simulink model "fig2"  (R2016b)
settings: Solver=VariableStepAuto  StartTime=0.0  StopTime=70  RelTol=1e-3
values from neighbouring files (symbols this model uses):
  c = 0.25    [Lab2.m]    (also in lab2.m)
  g = 9.81    [Lab2.m]    (also in lab2.m)
  l = 2    [Lab2.m]    (also in lab2.m)
  m = 1    [Lab2.m]    (also in lab2.m)
settings Model: Creator=ee105-abq  LastModifiedBy=ee105-abq

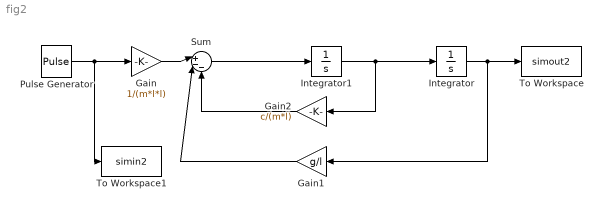
== system fig2 ==
  Gain : Gain  Gain=1/(m*l*l)
  Gain1 : Gain  Gain=g/l
  Gain2 : Gain  Gain=c/(m*l)
  Integrator : Integrator
  Integrator1 : Integrator
  Pulse Generator : DiscretePulseGenerator  PulseType=Time based  Amplitude=250  Period=100  PulseWidth=0.2
  Sum : Sum  Inputs=|+--
  To Workspace : ToWorkspace  VariableName=simout2  SaveFormat=Timeseries  SampleTime=-1
  To Workspace1 : ToWorkspace  VariableName=simin2  SaveFormat=Timeseries  SampleTime=-1
  wires:
  Gain/1 -> Sum/1
  Integrator/1 -> Gain1/1, To Workspace/1
  Gain1/1 -> Sum/2
  Gain2/1 -> Sum/3
  Sum/1 -> Integrator1/1
  Integrator1/1 -> Gain2/1, Integrator/1
  Pulse Generator/1 -> To Workspace1/1, Gain/1
